simulink model "p3ph_pll"  (Simulink 6.3)
settings: Solver=FixedStepDiscrete  SolverMode=SingleTasking  StartTime=0.0004  StopTime=12  RelTol=1e-3  AbsTol=1e-2
undefined symbols (not defined in the file or in its folder): DiscIntNeverNeededParam
libraries: powerlib_extras x3
settings Model: Creator=sybille  LastModifiedBy=priyesh  ExtModeTrigMode=oneshot  ExtModeArmWhenConnect=off  ExtModeAutoUpdateStatusClock=off  StrictBusMsg=None  ProdHWDeviceType=Specified
settings DataIOCC: Decimation=10  LimitDataPoints=off  SaveFinalState=on  SaveOutput=off  SignalLoggingName=sigsOut
settings OptimizationCC: BlockReduction=off  BooleanDataType=off  InlineInvariantSignals=on
settings DebuggingCC: CheckExecutionContextPreStartOutputMsg=on  CheckExecutionContextRuntimeOutputMsg=on  SolverPrmCheckMsg=none  UnconnectedInputMsg=none  UnconnectedOutputMsg=none
settings HardwareCC: ProdBitPerShort=32  ProdBitPerInt=16  ProdHWDeviceType=Specified  TargetUnknown=on
settings RTWCC: TemplateMakefile=grt_vc.tmf

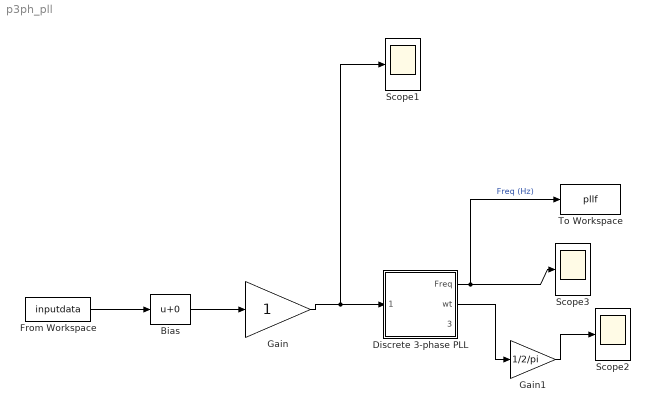
== system p3ph_pll ==
  Bias : Bias
  Discrete 3-phase PLL : Subsystem  AncestorBlock=|  mask(Discrete 3-phase PLL){Fmin=45, Par_Init=[0  50], ParK=[60 1400], Ts=1/2500}
      | powerlib_extras/Discrete 
      | Control Blocks/Discrete
      | 3-phase PLL
      mask prompts: Fmin "Minimum frequency (Hz):"; Par_Init "Initial inputs:[ Phase(degrees)   Frequency(Hz) ]"; ParK "Regulator gains [ Kp  Ki ]"; Ts "Sample time:"
      mask help:
      | This Phase Locked Loop (PLL) system can be used  to synchronize on a set of variable frequency, three-phase sinusoidal signals.
      |
      | Input 1: Vector containing the normalized
      |              three-phase signals [Va Vb Vc]
      | Output 1:  Measured frequency (Hz) = w/(2pi)
      | Output 2:  Ramp w.t   varying between  0 and 2*pi,
      | synchronized on zero crossings of the fundamental (positive-sequence) of phase A.
      | Output 3: Vector [sin(wt) cos(wt)]
      mask init:
      | Kp=ParK(1);
      | Ki=ParK(2);
      | Phase_Init=Par_Init(1);
      | Finit=Par_Init(2);
  From Workspace : FromWorkspace  VariableName=inputdata  SampleTime=1/2500  Interpolate=off  OutputAfterFinalValue=Setting to zero
  Gain : Gain
  Gain1 : Gain  Gain=1/2/pi  SaturateOnIntegerOverflow=on
  Scope1 : Scope
      settings: TimeRange=0.05  YMin=0.5  YMax=2.4  SaveName=ScopeData2  DataFormat=Array  SampleInput=on
  Scope2 : Scope
      settings: TimeRange=0.05  YMin=-1.1  YMax=1.1  DataFormat=Array  SampleInput=on
  Scope3 : Scope
      settings: TimeRange=0.05  YMin=-1.1  YMax=1.1  DataFormat=Array  SampleInput=on
  To Workspace : ToWorkspace  VariableName=pllf  SampleTime=-1  SaveFormat=Array
  wires:
  Gain1/1 -> Scope2/1
  Discrete 3-phase PLL/2(wt) -> Gain1/1
  Discrete 3-phase PLL/1(Freq) -> To Workspace/1, Scope3/1  "Freq (Hz)"
  Bias/1 -> Gain/1
  Gain/1 -> Discrete 3-phase PLL/1(Vabc (pu)), Scope1/1
  From Workspace/1 -> Bias/1

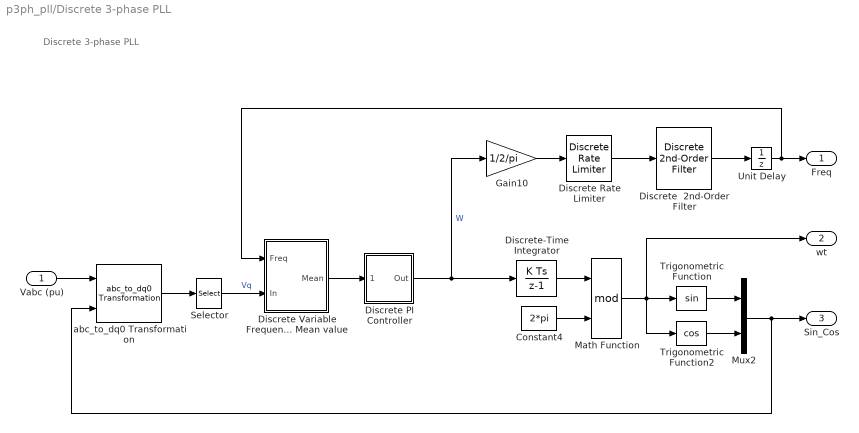
== system p3ph_pll/Discrete 3-phase PLL ==
  note: Discrete 3-phase PLL
  Vabc (pu) : Inport  PortDimensions=3
  Constant4 : Constant  Value=2*pi
  Discrete PI Controller : Subsystem  AncestorBlock=|  mask(Discrete PI Controller){Kp=Kp, Ki=Ki, Par_Limits=2*pi*Finit*[1.25 0.75], Init=2*pi*Finit, Ts=Ts}
      | powerlib_extras/Discrete 
      | Control Blocks/Discrete
      | PI Controller
      mask prompts: Kp "Proportional gain (Kp):"; Ki "Integral gain (Ki):"; Par_Limits "Output limits: [ Upper   Lower ]"; Init "Output initial value:"; Ts "Sample time:"
      mask help: This block implements a discrete PI controller.
      mask init:
      | UpperLimit=Par_Limits(1);
      | LowerLimit=Par_Limits(2);
      mask Display: disp('PI');
  Discrete Rate Limiter : powerlib_extras/Discrete  Control Blocks/Discrete Rate Limiter  R=12  F=-12  Vinit=Finit  Ts=Ts
  Discrete Variable Frequency Mean value : Subsystem  AncestorBlock=|  mask(Discrete Variable-Frequency Mean Value){Finit=Finit, Fmin=Fmin, Vinit=0, Ts=Ts}
      | powerlib_extras/Discrete
      | Measurements/Discrete
      | Variable Frequency
      | Mean value
      mask prompts: Finit "Initial frequency (Hz):"; Fmin "Minimum frequency (Hz):"; Vinit "Initial input (DC component):"; Ts "Sample time:"
      mask help:
      | This discrete block computes the mean value of the input signal (port In) over a running window of one cycle of a specified frequency (port Freq).
      |
      | For the first cycle of simulation (specified by the parameter "Initial frequency"), the ouput is held to the value of the  "Initial input" parameter.
      |
      | The value of the parameter "Minimum frequency" is used to determine the buffer size of the "Variable Transport Delay" block found inside this subsystem.
      mask init:
      | MaxDelay=1/Fmin+Ts;
  Discrete  2nd-Order Filter : powerlib_extras/Discrete  Control Blocks/Discrete  2nd-Order Filter  FilterType=Lowpass  Fo=25  Zeta=0.707  Ts=Ts  Initialize=on  Vac_Init=[0 0 Finit]  Vdc_Init=Finit  PlotResponse=off  param1=[1 500 0.1]
  Discrete-Time Integrator : DiscreteIntegrator  InitialCondition=Phase_Init*pi/180  SampleTime=Ts  ICPrevOutput=DiscIntNeverNeededParam  ICPrevScaledInput=DiscIntNeverNeededParam
  Gain10 : Gain  Gain=1/2/pi  SaturateOnIntegerOverflow=on
  Math Function : Math  Operator=mod  SaturateOnIntegerOverflow=on
  Mux2 : Mux  Inputs=2
  Selector : Selector  Elements=2  InputPortWidth=3
  Trigonometric Function : Trigonometry
  Trigonometric Function2 : Trigonometry  Operator=cos
  Unit Delay : UnitDelay  X0=Finit  SampleTime=Ts
  abc_to_dq0 Transformation : powerlib_extras/Measurements/abc_to_dq0 Transformation
  Freq : Outport
  wt : Outport  Port=2
  Sin_Cos : Outport  Port=3
  wires:
  Selector/1 -> Discrete Variable Frequency Mean value/2(In)  "Vq"
  Discrete  2nd-Order Filter/1 -> Unit Delay/1
  Unit Delay/1 -> Discrete Variable Frequency Mean value/1(Freq), Freq/1
  Discrete Rate Limiter/1 -> Discrete  2nd-Order Filter/1
  Gain10/1 -> Discrete Rate Limiter/1
  Discrete PI Controller/1(Out) -> Gain10/1, Discrete-Time Integrator/1  "W"
  Mux2/1 -> Sin_Cos/1, abc_to_dq0 Transformation/2
  Trigonometric Function2/1 -> Mux2/2
  Trigonometric Function/1 -> Mux2/1
  Math Function/1 -> wt/1, Trigonometric Function2/1, Trigonometric Function/1
  Discrete-Time Integrator/1 -> Math Function/1
  Constant4/1 -> Math Function/2
  abc_to_dq0 Transformation/1 -> Selector/1
  Vabc (pu)/1 -> abc_to_dq0 Transformation/1
  Discrete Variable Frequency Mean value/1(Mean) -> Discrete PI Controller/1(Error)

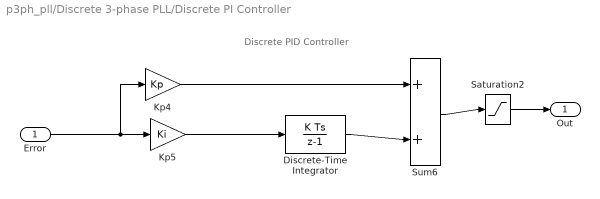
== system p3ph_pll/Discrete 3-phase PLL/Discrete PI Controller ==
  note: Discrete PID Controller
  Error : Inport
  Discrete-Time Integrator : DiscreteIntegrator  InitialCondition=Init  SampleTime=Ts  LimitOutput=on  UpperSaturationLimit=UpperLimit  LowerSaturationLimit=LowerLimit  ICPrevOutput=DiscIntNeverNeededParam  ICPrevScaledInput=DiscIntNeverNeededParam
  Kp4 : Gain  Gain=Kp  SaturateOnIntegerOverflow=on
  Kp5 : Gain  Gain=Ki  SaturateOnIntegerOverflow=on
  Saturation2 : Saturate  UpperLimit=UpperLimit  LowerLimit=LowerLimit
  Sum6 : Sum  SaturateOnIntegerOverflow=on  InputSameDT=on
  Out : Outport  InitialOutput=0
  wires:
  Saturation2/1 -> Out/1
  Discrete-Time Integrator/1 -> Sum6/2
  Kp4/1 -> Sum6/1
  Kp5/1 -> Discrete-Time Integrator/1
  Sum6/1 -> Saturation2/1
  Error/1 -> Kp5/1, Kp4/1

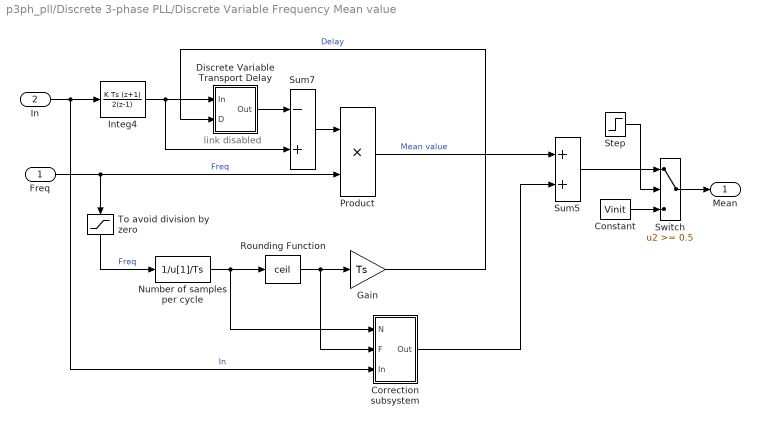
== system p3ph_pll/Discrete 3-phase PLL/Discrete Variable Frequency Mean value ==
  note: link disabled
  Freq : Inport  PortDimensions=1
  In : Inport  Port=2  PortDimensions=1
  Constant : Constant  Value=Vinit
  Correction subsystem : Subsystem
  Discrete Variable Transport Delay : Subsystem  AncestorBlock=|  mask(Discrete variable transport delay){MaxDelay=MaxDelay, InitialValue=0, Ts=Ts}
      | powerlib_extras/Discrete 
      | Control Blocks/Discrete Variable
      | Transport Delay
      mask prompts: MaxDelay "Maximum delay (s):"; InitialValue "Initial input:"; Ts "Sample time:"
      mask help:
      | Apply a delay to the first input (In) signal.
      | The second input (D) specifies the delay time.
  Gain : Gain  Gain=Ts  SaturateOnIntegerOverflow=on
  Integ4 : DiscreteIntegrator  IntegratorMethod=Integration: Trapezoidal  SampleTime=Ts  ICPrevOutput=DiscIntNeverNeededParam  ICPrevScaledInput=DiscIntNeverNeededParam
  Number of samples per cycle : Fcn  Expr=1/u[1]/Ts
  Product : Product  SaturateOnIntegerOverflow=on  InputSameDT=on
  Rounding Function : Rounding  Operator=ceil
  Step : Step  Time=1/Finit  SampleTime=Ts
  Sum5 : Sum  SaturateOnIntegerOverflow=on  InputSameDT=on
  Sum7 : Sum  Inputs=-+  SaturateOnIntegerOverflow=on  InputSameDT=on
  Switch : Switch  Threshold=0.5  InputSameDT=on
  To avoid division by zero : Saturate  Orientation=down  UpperLimit=1e6  LowerLimit=1e-6
  Mean : Outport
  wires:
  In/1 -> Integ4/1, Correction subsystem/3(In)  "In"
  Product/1 -> Sum5/1  "Mean value"
  Discrete Variable Transport Delay/1(Out) -> Sum7/1
  Sum7/1 -> Product/1
  Integ4/1 -> Discrete Variable Transport Delay/1(In), Sum7/2
  Freq/1 -> Product/2, To avoid division by zero/1  "Freq"
  Gain/1 -> Discrete Variable Transport Delay/2(D)  "Delay"
  Rounding Function/1 -> Gain/1, Correction subsystem/2(F)
  Number of samples per cycle/1 -> Rounding Function/1, Correction subsystem/1(N)
  Sum5/1 -> Switch/1
  Constant/1 -> Switch/3
  Switch/1 -> Mean/1
  To avoid division by zero/1 -> Number of samples per cycle/1  "Freq"
  Correction subsystem/1(Out) -> Sum5/2
  Step/1 -> Switch/2

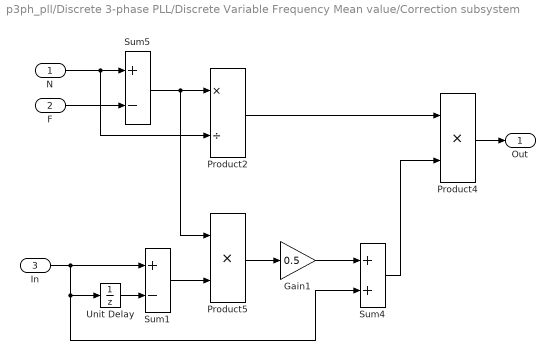
== system p3ph_pll/Discrete 3-phase PLL/Discrete Variable Frequency Mean value/Correction subsystem ==
  N : Inport
  F : Inport  Port=2
  In : Inport  Port=3
  Gain1 : Gain  Gain=0.5  SaturateOnIntegerOverflow=on
  Product2 : Product  Inputs=*/  SaturateOnIntegerOverflow=on  InputSameDT=on
  Product4 : Product  Inputs=**  SaturateOnIntegerOverflow=on  InputSameDT=on
  Product5 : Product  Inputs=**  SaturateOnIntegerOverflow=on  InputSameDT=on
  Sum1 : Sum  Inputs=+-  SaturateOnIntegerOverflow=on  InputSameDT=on
  Sum4 : Sum  SaturateOnIntegerOverflow=on  InputSameDT=on
  Sum5 : Sum  Inputs=+-  SaturateOnIntegerOverflow=on  InputSameDT=on
  Unit Delay : UnitDelay  SampleTime=Ts
  Out : Outport
  wires:
  Unit Delay/1 -> Sum1/2
  N/1 -> Sum5/1, Product2/2
  F/1 -> Sum5/2
  Sum5/1 -> Product2/1, Product5/1
  Product2/1 -> Product4/1
  In/1 -> Sum1/1, Unit Delay/1, Sum4/2
  Sum1/1 -> Product5/2
  Product5/1 -> Gain1/1
  Gain1/1 -> Sum4/1
  Sum4/1 -> Product4/2
  Product4/1 -> Out/1

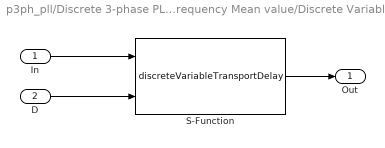
== system p3ph_pll/Discrete 3-phase PLL/Discrete Variable Frequency Mean value/Discrete Variable Transport Delay ==
  In : Inport
  D : Inport  Port=2
  "S-Function " : S-Function  FunctionName=discreteVariableTransportDelay  Parameters=MaxDelay,Ts,InitialValue
  Out : Outport
  wires:
  "S-Function "/1 -> Out/1
  In/1 -> "S-Function "/1
  D/1 -> "S-Function "/2
